simulink model "Thirteenlevel"  (R2023b)
settings: Solver=ode23tb  StartTime=0.0  StopTime=0.3  RelTol=1e-3  EnableMultiTasking=on
libraries: spsDiodeLib x8, spsIGBTDiodeLib x8, spsSeriesRLCBranchLib x7, spsVoltageMeasurementLib x5, spsDCVoltageSourceLib x2, sps_lib x1
settings Model: Creator=Dharma  LastModifiedBy=User
settings SolverCC: ZeroCrossControl=DisableAll  AlgebraicLoopSolver=TrustRegion
settings DataIOCC: LimitDataPoints=on  SaveFormat=Array  SignalLoggingSaveFormat=ModelDataLogs  ReturnWorkspaceOutputs=off
settings OptimizationCC: ExpressionDepthLimit=2147483647  LifeSpan=inf
settings DebuggingCC: UnderspecifiedInitializationDetection=Classic  MergeDetectMultiDrivingBlocksExec=none  SolverPrmCheckMsg=warning  FcnCallInpInsideContextMsg=warning  UnconnectedInputMsg=warning  UnconnectedOutputMsg=warning  UnconnectedLineMsg=warning  StateNameClashWarn=warning  SFUnexpectedBacktrackingDiag=warning  SFNoUnconditionalDefaultTransitionDiag=warning  SFExecutionAtInitializationDiag=none  ArithmeticOperatorsInVariantConditions=warning
settings HardwareCC: ProdBitPerPointer=32  ProdBitPerSizeT=32  ProdBitPerPtrDiffT=32  ProdLargestAtomicFloat=None  ProdIntDivRoundTo=Undefined  ProdEndianess=Unspecified  ProdWordSize=32  ProdHWDeviceType=32-bit Generic
settings ModelReferenceCC: PropagateSignalLabelsOutOfModel=off
settings SFSimCC: SimUseLocalCustomCode=off  CustomCodeUndefinedFunction=UseInterfaceOnly
settings RTWCC: RTWUseLocalCustomCode=off
settings CodeAppCC: StateflowObjectComments=on
settings GRTTargetCC: TargetLangStandard=C89/C90 (ANSI)  CombineOutputUpdateFcns=off  GRTInterface=on
settings ConfigComp: CovMetricSettings=dw  CovSaveCumulativeToWorkspaceVar=on  CovSaveSingleToWorkspaceVar=on  CovExternalEMLEnable=off
settings SimscapeCC: SimscapeNormalizeSystem=off

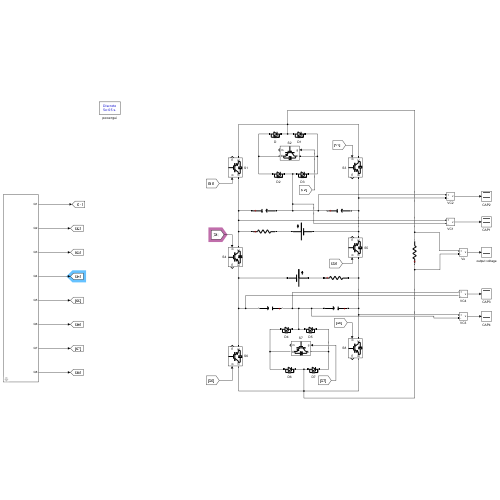
[thumbnail: Simulink's stored preview of the top-level diagram]
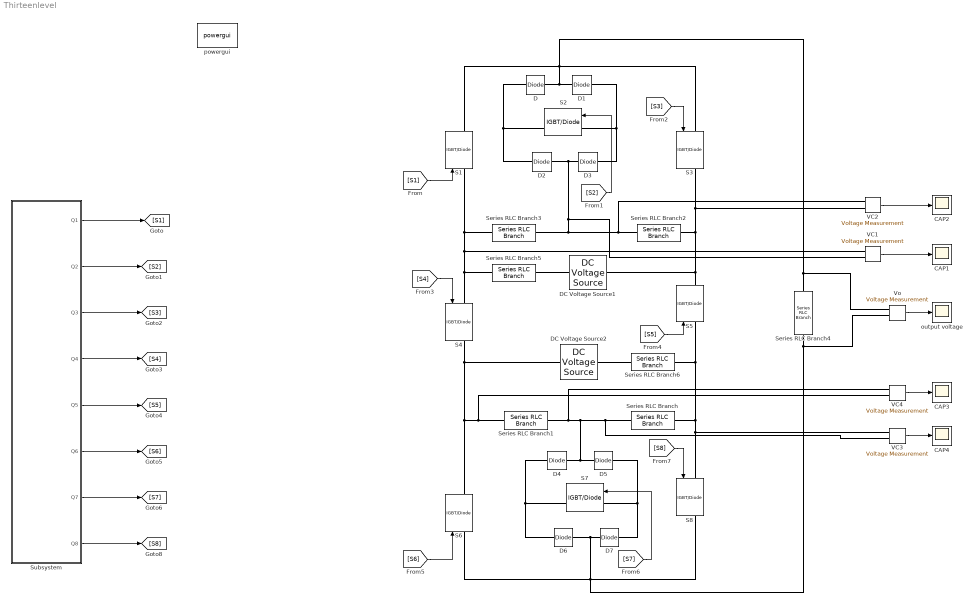
== system Thirteenlevel ==
  CAP{1..4} (4 alike) : Scope
  D{,1..7} (8 alike) : spsDiodeLib/Diode  Ron=0.001  Lon=0  Vf=0.8  IC=0  UseSnubber=off  Rs=500  Cs=250e-9  Measurements=off
  DC Voltage Source1 : spsDCVoltageSourceLib/DC Voltage Source  Amplitude=100  Measurements=None
  DC Voltage Source2 : spsDCVoltageSourceLib/DC Voltage Source  Amplitude=200  Measurements=None
  S{1..8} (8 alike) : spsIGBTDiodeLib/IGBT//Diode  Ron=1e-3  Rs=1e5  Cs=inf  Measurements=on
  Series RLC Branch : spsSeriesRLCBranchLib/Series RLC Branch  LConnTagsString=__new0  RConnTagsString=__new0  BranchType=C  Resistance=12  Inductance=1e-3  SetiL0=off  InitialCurrent=0  Capacitance=1000e-6  Setx0=on  InitialVoltage=100  Measurements=None
  Series RLC Branch1 : spsSeriesRLCBranchLib/Series RLC Branch  LConnTagsString=__new0  RConnTagsString=__new0  BranchType=C  Resistance=12  Inductance=1e-3  SetiL0=off  InitialCurrent=0  Capacitance=1000e-6  Setx0=on  InitialVoltage=100  Measurements=None
  Series RLC Branch2 : spsSeriesRLCBranchLib/Series RLC Branch  LConnTagsString=__new0  RConnTagsString=__new0  BranchType=C  Resistance=12  Inductance=1e-3  SetiL0=off  InitialCurrent=0  Capacitance=1000e-6  Setx0=on  InitialVoltage=50  Measurements=None
  Series RLC Branch3 : spsSeriesRLCBranchLib/Series RLC Branch  LConnTagsString=__new0  RConnTagsString=__new0  BranchType=C  Resistance=12  Inductance=1e-3  SetiL0=off  InitialCurrent=0  Capacitance=1000e-6  Setx0=on  InitialVoltage=50  Measurements=None
  Series RLC Branch4 : spsSeriesRLCBranchLib/Series RLC Branch  LConnTagsString=__new0  RConnTagsString=__new0  BranchType=R  Resistance=100  Inductance=1e-3  SetiL0=off  InitialCurrent=0  Capacitance=1e-6  Setx0=off  InitialVoltage=0  Measurements=None
  Series RLC Branch5 : spsSeriesRLCBranchLib/Series RLC Branch  LConnTagsString=__new0  RConnTagsString=__new0  BranchType=R  Resistance=1e-3  Inductance=1e-3  SetiL0=off  InitialCurrent=0  Capacitance=1e-6  Setx0=off  InitialVoltage=0  Measurements=None
  Series RLC Branch6 : spsSeriesRLCBranchLib/Series RLC Branch  LConnTagsString=__new0  RConnTagsString=__new0  BranchType=R  Resistance=1e-3  Inductance=1e-3  SetiL0=off  InitialCurrent=0  Capacitance=1e-6  Setx0=off  InitialVoltage=0  Measurements=None
  Subsystem : Subsystem  mask{freq=50}
      mask prompts: freq "frequency"
  VC{1..4} (4 alike) : spsVoltageMeasurementLib/Voltage Measurement  PhasorSimulation=off  OutputType=Complex  PSBequivalent=0
  Vo : spsVoltageMeasurementLib/Voltage Measurement  PhasorSimulation=off  OutputType=Complex  PSBequivalent=0
  output voltage : Scope
  powergui : sps_lib/powergui  Priority=1  SimulationMode=Discrete  SampleTime=50e-6  frequency=60  Iterations=50  frequencyindice=0  Pbase=100e6  ErrMax=1e-4  UnitsV=kV  UnitsW=MW  buscounter=0  FunctionMessages=off  echomessages=off  EnableUseOfTLC=off  CurrentSourceSwitches=off  DisableSnubberDevices=off  DisableRonSwitches=off  DisableVfSwitches=off  DisplayEquations=off  AutomaticDiscreteSolvers=off  SolverType=Tustin  Interpol=off  ExternalGateDelay=off  methode=off  Ts=0  x0status=blocks  SPID=off  SwTol=0  HookPort=off  NonlinearTolerance=1e-4  nMaxIteration=100  ContinueOnMaxIteration=off  RestoreLinks=warning  ResistiveCurrentMeasurement=off  Frange=[0:2:500]  Ylog=off  Xlog=on  ShowGrid=off  save=off  variable=ZData  structure=simout  ZoomFFT=off  StartTime=0.0  cycles=20  DisplayStyle=1  fundamental=50  FreqAxis=on  MaxFrequency=1000  frequencyindicesteady=1  RmsSteady=1  display=off
  wires:
  [S1] -> S1/1
  [S2] -> S2/1
  [S3] -> S3/1
  [S4] -> S4/1
  [S5] -> S5/1
  [S6] -> S6/1
  [S7] -> S7/1
  [S8] -> S8/1
  Subsystem/1(Q1) -> [S1]
  Subsystem/2(Q2) -> [S2]
  Subsystem/3(Q3) -> [S3]
  Subsystem/4(Q4) -> [S4]
  Subsystem/5(Q5) -> [S5]
  Subsystem/6(Q6) -> [S6]
  Subsystem/7(Q7) -> [S7]
  Subsystem/8(Q8) -> [S8]
  Vo/1 -> output voltage/1
  VC1/1 -> CAP1/1
  VC2/1 -> CAP2/1
  VC3/1 -> CAP4/1
  VC4/1 -> CAP3/1
  connections:
  D5/LConn1 -- VC4/LConn1 -- Series RLC Branch1/LConn1 -- VC3/LConn2 -- Series RLC Branch/RConn1 -- D4/RConn1
  S5/LConn1 -- Series RLC Branch6/RConn1 -- VC3/LConn1 -- S8/LConn1 -- Series RLC Branch/LConn1
  DC Voltage Source2/LConn1 -- S6/RConn1 -- VC4/LConn2 -- Series RLC Branch1/RConn1 -- S4/RConn1
  S4/LConn1 -- Series RLC Branch5/LConn1 -- Series RLC Branch3/LConn1 -- S1/LConn1 -- VC1/LConn1
  DC Voltage Source1/LConn1 -- S5/RConn1 -- VC2/LConn2 -- S3/RConn1 -- Series RLC Branch2/RConn1
  D3/LConn1 -- VC2/LConn1 -- Series RLC Branch2/LConn1 -- Series RLC Branch3/RConn1 -- VC1/LConn2 -- D2/RConn1
  D1/RConn1 -- S2/LConn1 -- D3/RConn1
  D2/LConn1 -- S2/RConn1 -- D/LConn1
  D7/LConn1 -- D6/RConn1 -- Series RLC Branch4/LConn1 -- Vo/LConn2 -- S8/RConn1 -- S6/LConn1
  D5/RConn1 -- S7/LConn1 -- D7/RConn1
  D6/LConn1 -- S7/RConn1 -- D4/LConn1
  D/RConn1 -- S3/LConn1 -- Vo/LConn1 -- Series RLC Branch4/RConn1 -- S1/RConn1 -- D1/LConn1
  Series RLC Branch5/RConn1 -- DC Voltage Source1/RConn1
  Series RLC Branch6/LConn1 -- DC Voltage Source2/RConn1

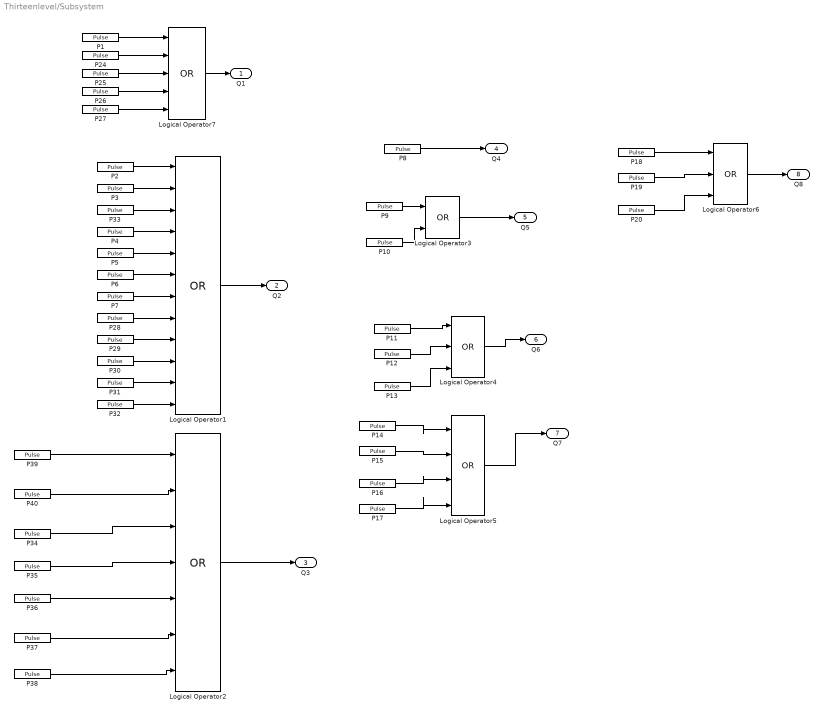
== system Thirteenlevel/Subsystem ==
  Logical Operator1 : Logic  Operator=OR  Inputs=12  IconShape=distinctive  AllPortsSameDT=off  OutDataTypeStr=boolean
  Logical Operator2 : Logic  Operator=OR  Inputs=7  IconShape=distinctive  AllPortsSameDT=off  OutDataTypeStr=boolean
  Logical Operator3 : Logic  Operator=OR  IconShape=distinctive  AllPortsSameDT=off  OutDataTypeStr=boolean
  Logical Operator4 : Logic  Operator=OR  Inputs=3  IconShape=distinctive  AllPortsSameDT=off  OutDataTypeStr=boolean
  Logical Operator5 : Logic  Operator=OR  Inputs=4  IconShape=distinctive  AllPortsSameDT=off  OutDataTypeStr=boolean
  Logical Operator6 : Logic  Operator=OR  Inputs=3  IconShape=distinctive  AllPortsSameDT=off  OutDataTypeStr=boolean
  Logical Operator7 : Logic  Operator=OR  Inputs=5  IconShape=distinctive  AllPortsSameDT=off  OutDataTypeStr=boolean
  P1 : DiscretePulseGenerator  PulseType=Time based  Period=1/freq  PulseWidth=(100/24)  PhaseDelay=((1/freq)/24)
  P10 : DiscretePulseGenerator  PulseType=Time based  Period=1/freq  PulseWidth=(100/24)  PhaseDelay=((1/freq)/24)*23
  P11 : DiscretePulseGenerator  PulseType=Time based  Period=1/freq  PulseWidth=(100/24)*5  PhaseDelay=((1/freq)/24)*3
  P12 : DiscretePulseGenerator  PulseType=Time based  Period=1/freq  PulseWidth=(100/24)*2  PhaseDelay=((1/freq)/24)*12
  P13 : DiscretePulseGenerator  PulseType=Time based  Period=1/freq  PulseWidth=(100/24)*2  PhaseDelay=((1/freq)/24)*21
  P14 : DiscretePulseGenerator  PulseType=Time based  Period=1/freq  PulseWidth=(100/24)  PhaseDelay=((1/freq)/24)*2
  P15 : DiscretePulseGenerator  PulseType=Time based  Period=1/freq  PulseWidth=(100/24)  PhaseDelay=((1/freq)/24)*8
  P16 : DiscretePulseGenerator  PulseType=Time based  Period=1/freq  PulseWidth=(100/24)  PhaseDelay=((1/freq)/24)*14
  P17 : DiscretePulseGenerator  PulseType=Time based  Period=1/freq  PulseWidth=(100/24)  PhaseDelay=((1/freq)/24)*20
  P18 : DiscretePulseGenerator  PulseType=Time based  Period=1/freq  PulseWidth=(100/24)*2
  P19 : DiscretePulseGenerator  PulseType=Time based  Period=1/freq  PulseWidth=(100/24)*3  PhaseDelay=((1/freq)/24)*9
  P2 : DiscretePulseGenerator  PulseType=Time based  Period=1/freq  PulseWidth=(100/24)
  P20 : DiscretePulseGenerator  PulseType=Time based  Period=1/freq  PulseWidth=(100/24)*5  PhaseDelay=((1/freq)/24)*15
  P24 : DiscretePulseGenerator  PulseType=Time based  Period=1/freq  PulseWidth=(100/24)  PhaseDelay=((1/freq)/24)*5
  P25 : DiscretePulseGenerator  PulseType=Time based  Period=1/freq  PulseWidth=(100/24)  PhaseDelay=((1/freq)/24)*9
  P26 : DiscretePulseGenerator  PulseType=Time based  Period=1/freq  PulseWidth=(100/24)  PhaseDelay=((1/freq)/24)*15
  P27 : DiscretePulseGenerator  PulseType=Time based  Period=1/freq  PulseWidth=(100/24)  PhaseDelay=((1/freq)/24)*19
  P28 : DiscretePulseGenerator  PulseType=Time based  Period=1/freq  PulseWidth=(100/24)  PhaseDelay=((1/freq)/24)*14
  P29 : DiscretePulseGenerator  PulseType=Time based  Period=1/freq  PulseWidth=(100/24)  PhaseDelay=((1/freq)/24)*16
  P3 : DiscretePulseGenerator  PulseType=Time based  Period=1/freq  PulseWidth=(100/24)  PhaseDelay=((1/freq)/24)*2
  P30 : DiscretePulseGenerator  PulseType=Time based  Period=1/freq  PulseWidth=(100/24)  PhaseDelay=((1/freq)/24)*18
  P31 : DiscretePulseGenerator  PulseType=Time based  Period=1/freq  PulseWidth=(100/24)  PhaseDelay=((1/freq)/24)*20
  P32 : DiscretePulseGenerator  PulseType=Time based  Period=1/freq  PulseWidth=(100/24)  PhaseDelay=((1/freq)/24)*22
  P33 : DiscretePulseGenerator  PulseType=Time based  Period=1/freq  PulseWidth=(100/24)  PhaseDelay=((1/freq)/24)*4
  P34 : DiscretePulseGenerator  PulseType=Time based  Period=1/freq  PulseWidth=(100/24)  PhaseDelay=((1/freq)/24)*11
  P35 : DiscretePulseGenerator  PulseType=Time based  Period=1/freq  PulseWidth=(100/24)  PhaseDelay=((1/freq)/24)*13
  P36 : DiscretePulseGenerator  PulseType=Time based  Period=1/freq  PulseWidth=(100/24)  PhaseDelay=((1/freq)/24)*17
  P37 : DiscretePulseGenerator  PulseType=Time based  Period=1/freq  PulseWidth=(100/24)  PhaseDelay=((1/freq)/24)*21
  P38 : DiscretePulseGenerator  PulseType=Time based  Period=1/freq  PulseWidth=(100/24)  PhaseDelay=((1/freq)/24)*23
  P39 : DiscretePulseGenerator  PulseType=Time based  Period=1/freq  PulseWidth=(100/24)  PhaseDelay=((1/freq)/24)*3
  P4 : DiscretePulseGenerator  PulseType=Time based  Period=1/freq  PulseWidth=(100/24)  PhaseDelay=((1/freq)/24)*6
  P40 : DiscretePulseGenerator  PulseType=Time based  Period=1/freq  PulseWidth=(100/24)  PhaseDelay=((1/freq)/24)*7
  P5 : DiscretePulseGenerator  PulseType=Time based  Period=1/freq  PulseWidth=(100/24)  PhaseDelay=((1/freq)/24)*8
  P6 : DiscretePulseGenerator  PulseType=Time based  Period=1/freq  PulseWidth=(100/24)  PhaseDelay=((1/freq)/24)*10
  P7 : DiscretePulseGenerator  PulseType=Time based  Period=1/freq  PulseWidth=(100/24)  PhaseDelay=((1/freq)/24)*12
  P8 : DiscretePulseGenerator  PulseType=Time based  Period=1/freq  PulseWidth=(100/24)*11  PhaseDelay=((1/freq)/24)*12
  P9 : DiscretePulseGenerator  PulseType=Time based  Period=1/freq  PulseWidth=(100/24)*12
  Q1 : Outport
  Q2 : Outport  Port=2
  Q3 : Outport  Port=3
  Q4 : Outport  Port=4
  Q5 : Outport  Port=5
  Q6 : Outport  Port=6
  Q7 : Outport  Port=7
  Q8 : Outport  Port=8
  wires:
  P8/1 -> Q4/1
  Logical Operator7/1 -> Q1/1
  P1/1 -> Logical Operator7/1
  P27/1 -> Logical Operator7/5
  P26/1 -> Logical Operator7/4
  P24/1 -> Logical Operator7/2
  P25/1 -> Logical Operator7/3
  Logical Operator1/1 -> Q2/1
  P2/1 -> Logical Operator1/1
  P33/1 -> Logical Operator1/3
  P3/1 -> Logical Operator1/2
  P4/1 -> Logical Operator1/4
  P5/1 -> Logical Operator1/5
  P6/1 -> Logical Operator1/6
  P7/1 -> Logical Operator1/7
  P28/1 -> Logical Operator1/8
  P29/1 -> Logical Operator1/9
  P30/1 -> Logical Operator1/10
  P31/1 -> Logical Operator1/11
  P32/1 -> Logical Operator1/12
  Logical Operator2/1 -> Q3/1
  P38/1 -> Logical Operator2/7
  P36/1 -> Logical Operator2/5
  P37/1 -> Logical Operator2/6
  P40/1 -> Logical Operator2/2
  P39/1 -> Logical Operator2/1
  P35/1 -> Logical Operator2/4
  P34/1 -> Logical Operator2/3
  Logical Operator3/1 -> Q5/1
  P9/1 -> Logical Operator3/1
  P10/1 -> Logical Operator3/2
  Logical Operator4/1 -> Q6/1
  P11/1 -> Logical Operator4/1
  P12/1 -> Logical Operator4/2
  P13/1 -> Logical Operator4/3
  P15/1 -> Logical Operator5/2
  P14/1 -> Logical Operator5/1
  P16/1 -> Logical Operator5/3
  P17/1 -> Logical Operator5/4
  Logical Operator5/1 -> Q7/1
  Logical Operator6/1 -> Q8/1
  P18/1 -> Logical Operator6/1
  P19/1 -> Logical Operator6/2
  P20/1 -> Logical Operator6/3
